simulink model "MainSim"  (R2024a)
settings: Solver=ode4  StartTime=0.0  StopTime=simtime  FixedStep=0.1  RelTol=1e-3
values from neighbouring files (symbols this model uses):
  C = [1 0 0 0 0 0 -1 0 0 0 0 0 ... (45 elements, 5x9)]    [C.mat]
undefined symbols (not defined in the file or in its folder): Ki, Kp, ssest, syys, utrim, xtrim
libraries: neural x680
(part 4 of 12)

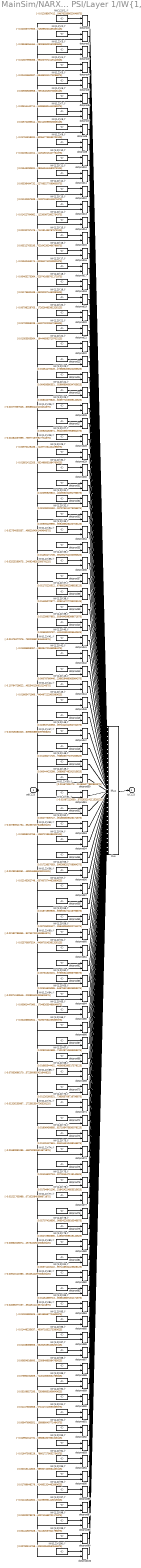
== system MainSim/NARX Controller NO PSI/Layer 1/IW{1,2} ==
  "pd{1,2}" : Inport  PortDimensions=5  SampleTime=0.1
      mask Display: e = 0.06;c1 = [120 230 180]/255;c2 = ([120 230 180]+0)/(256+128);c3 = ([120 230 180]+128)/(256+128);patch([0 1 1 0],[0 0 1 1],c1);patch([0 1 1 1-e 1-e 0+e],[0 0 1 1-e 0+e 0+e],c2);patch([0 0 1 1-e 0+e 0+e],[0 1 1 1-e 1-e 0+e],c3);plot([0 1 1 0 0],[0 0 1 1 0]);
  "IW{1,2}(1,:)'" : Constant  Value=[-0.012085674124014282593275737553994986228644847869873046875;-0.006873434973601206914028960426321646082215011119842529296875;-0.03332932307240245306534376368290395475924015045166015625;-0.03433322519643809689338098678490496240556240081787109375;0.030870812178684474413881133614268037490546703338623046875]
      mask Display: e = 0.06;c1 = [120 150 230]/255;c2 = ([120 150 230]+0)/383;c3 = ([120 150 230]+128)/383;patch([0 1 1 0],[0 0 1 1],c1);patch([0 1 1 1-e 1-e 0+e],[0 0 1 1-e 0+e 0+e],c2);patch([0 0 1 1-e 0+e 0+e],[0 1 1 1-e 1-e 0+e],c3);plot([0 1 1 0 0],[0 0 1 1 0]);disp('Weights');
  "IW{1,2}(10,:)'" : Constant  Value=[-0.022334120114864512707253396683881874196231365203857421875;0.03401133169790999943860043686072458513081073760986328125;-0.0140961839759349873146820897318320930935442447662353515625;-0.0105321300412540945490302846110353129915893077850341796875;0.0146962613745357205397024102921932353638112545013427734375]
      mask Display: e = 0.06;c1 = [120 150 230]/255;c2 = ([120 150 230]+0)/383;c3 = ([120 150 230]+128)/383;patch([0 1 1 0],[0 0 1 1],c1);patch([0 1 1 1-e 1-e 0+e],[0 0 1 1-e 0+e 0+e],c2);patch([0 0 1 1-e 0+e 0+e],[0 1 1 1-e 1-e 0+e],c3);plot([0 1 1 0 0],[0 0 1 1 0]);disp('Weights');
  "IW{1,2}(100,:)'" : Constant  Value=[0.007805117685184641100615277053975660237483680248260498046875;-0.016738192143750614537811571835845825262367725372314453125;0.0305525637743539746349341612585703842341899871826171875;0.02995618865728581770024874231239664368331432342529296875;-0.029207083950386396320464399423144641332328319549560546875]
      mask Display: e = 0.06;c1 = [120 150 230]/255;c2 = ([120 150 230]+0)/383;c3 = ([120 150 230]+128)/383;patch([0 1 1 0],[0 0 1 1],c1);patch([0 1 1 1-e 1-e 0+e],[0 0 1 1-e 0+e 0+e],c2);patch([0 0 1 1-e 0+e 0+e],[0 1 1 1-e 1-e 0+e],c3);plot([0 1 1 0 0],[0 0 1 1 0]);disp('Weights');
  "IW{1,2}(11,:)'" : Constant  Value=[0.0154329083187489911332956893375012441538274288177490234375;-0.022986085536823797070837827050127089023590087890625;0.024814779155320133841033936050735064782202243804931640625;0.0231971824718188550373820788763623568229377269744873046875;-0.0243675210208365751463066573023752425797283649444580078125]
      mask Display: e = 0.06;c1 = [120 150 230]/255;c2 = ([120 150 230]+0)/383;c3 = ([120 150 230]+128)/383;patch([0 1 1 0],[0 0 1 1],c1);patch([0 1 1 1-e 1-e 0+e],[0 0 1 1-e 0+e 0+e],c2);patch([0 0 1 1-e 0+e 0+e],[0 1 1 1-e 1-e 0+e],c3);plot([0 1 1 0 0],[0 0 1 1 0]);disp('Weights');
  "IW{1,2}(12,:)'" : Constant  Value=[0.005364947322163394170801975491258417605422437191009521484375;-0.0112431095377618119057760992518524290062487125396728515625;0.03357479632188732632247507581269019283354282379150390625;0.033744156754611308313140938253127387724816799163818359375;-0.031764486089429853910015566498259431682527065277099609375]
      mask Display: e = 0.06;c1 = [120 150 230]/255;c2 = ([120 150 230]+0)/383;c3 = ([120 150 230]+128)/383;patch([0 1 1 0],[0 0 1 1],c1);patch([0 1 1 1-e 1-e 0+e],[0 0 1 1-e 0+e 0+e],c2);patch([0 0 1 1-e 0+e 0+e],[0 1 1 1-e 1-e 0+e],c3);plot([0 1 1 0 0],[0 0 1 1 0]);disp('Weights');
  "IW{1,2}(13,:)'" : Constant  Value=[0.011323576395817040729507851892776670865714550018310546875;-0.0160785944939652557239551100565222441218793392181396484375;0.0287434696253211739713773198445778689347207546234130859375;0.0279514119935516079651360854541053413413465023040771484375;-0.0275897150154243812891774467743744025938212871551513671875]
      mask Display: e = 0.06;c1 = [120 150 230]/255;c2 = ([120 150 230]+0)/383;c3 = ([120 150 230]+128)/383;patch([0 1 1 0],[0 0 1 1],c1);patch([0 1 1 1-e 1-e 0+e],[0 0 1 1-e 0+e 0+e],c2);patch([0 0 1 1-e 0+e 0+e],[0 1 1 1-e 1-e 0+e],c3);plot([0 1 1 0 0],[0 0 1 1 0]);disp('Weights');
  "IW{1,2}(14,:)'" : Constant  Value=[-0.0142278498231365631288003470444891718216240406036376953125;-0.0098485858989617001968408516177078126929700374603271484375;-0.032202423742523557381733922966304817236959934234619140625;-0.03325848380519517977216281678920495323836803436279296875;0.029775514742350593644371059554032399319112300872802734375]
      mask Display: e = 0.06;c1 = [120 150 230]/255;c2 = ([120 150 230]+0)/383;c3 = ([120 150 230]+128)/383;patch([0 1 1 0],[0 0 1 1],c1);patch([0 1 1 1-e 1-e 0+e],[0 0 1 1-e 0+e 0+e],c2);patch([0 0 1 1-e 0+e 0+e],[0 1 1 1-e 1-e 0+e],c3);plot([0 1 1 0 0],[0 0 1 1 0]);disp('Weights');
  "IW{1,2}(15,:)'" : Constant  Value=[0.0223276747640495376590052956089493818581104278564453125;0.0284561503012705600823561979950682143680751323699951171875;0.02904798645340199436670758359468891285359859466552734375;0.0305503870117409294382415652080453583039343357086181640625;-0.0259989639895998880803063002531416714191436767578125]
      mask Display: e = 0.06;c1 = [120 150 230]/255;c2 = ([120 150 230]+0)/383;c3 = ([120 150 230]+128)/383;patch([0 1 1 0],[0 0 1 1],c1);patch([0 1 1 1-e 1-e 0+e],[0 0 1 1-e 0+e 0+e],c2);patch([0 0 1 1-e 0+e 0+e],[0 1 1 1-e 1-e 0+e],c3);plot([0 1 1 0 0],[0 0 1 1 0]);disp('Weights');
  "IW{1,2}(16,:)'" : Constant  Value=[0.005127631958366886399947048857939080335199832916259765625;0.00947650558097157778847385856124674319289624691009521484375;-0.0404557009729242522677594706692616455256938934326171875;-0.041547997688944203475980287976199178956449031829833984375;0.03786523265411989580542240219074301421642303466796875]
      mask Display: e = 0.06;c1 = [120 150 230]/255;c2 = ([120 150 230]+0)/383;c3 = ([120 150 230]+128)/383;patch([0 1 1 0],[0 0 1 1],c1);patch([0 1 1 1-e 1-e 0+e],[0 0 1 1-e 0+e 0+e],c2);patch([0 0 1 1-e 0+e 0+e],[0 1 1 1-e 1-e 0+e],c3);plot([0 1 1 0 0],[0 0 1 1 0]);disp('Weights');
  "IW{1,2}(17,:)'" : Constant  Value=[-0.0194245317476195757111501194458469399251043796539306640625;0.017930787047602224359987843627095571719110012054443359375;-0.01082284320194641484558228938794854911975562572479248046875;-0.009279432063260963092776734129074611701071262359619140625;0.01093748533229130064092782248508228803984820842742919921875]
      mask Display: e = 0.06;c1 = [120 150 230]/255;c2 = ([120 150 230]+0)/383;c3 = ([120 150 230]+128)/383;patch([0 1 1 0],[0 0 1 1],c1);patch([0 1 1 1-e 1-e 0+e],[0 0 1 1-e 0+e 0+e],c2);patch([0 0 1 1-e 0+e 0+e],[0 1 1 1-e 1-e 0+e],c3);plot([0 1 1 0 0],[0 0 1 1 0]);disp('Weights');
  "IW{1,2}(18,:)'" : Constant  Value=[-0.004632733645585514724307696354799190885387361049652099609375;0.038132997508550599274901315993702155537903308868408203125;-0.027774570134460885295624166246852837502956390380859375;-0.0258087635385522186359796847909819916822016239166259765625;0.0275425986452899444756337032913506845943629741668701171875]
      mask Display: e = 0.06;c1 = [120 150 230]/255;c2 = ([120 150 230]+0)/383;c3 = ([120 150 230]+128)/383;patch([0 1 1 0],[0 0 1 1],c1);patch([0 1 1 1-e 1-e 0+e],[0 0 1 1-e 0+e 0+e],c2);patch([0 0 1 1-e 0+e 0+e],[0 1 1 1-e 1-e 0+e],c3);plot([0 1 1 0 0],[0 0 1 1 0]);disp('Weights');
  "IW{1,2}(19,:)'" : Constant  Value=[0.0117563243958725520410535381188310566358268260955810546875;0.0199784928711961538849717356924884370528161525726318359375;0.035521756938338443221336859778602956794202327728271484375;0.037526953635152134058916573167152819223701953887939453125;-0.032272748785357442680155060088509344495832920074462890625]
      mask Display: e = 0.06;c1 = [120 150 230]/255;c2 = ([120 150 230]+0)/383;c3 = ([120 150 230]+128)/383;patch([0 1 1 0],[0 0 1 1],c1);patch([0 1 1 1-e 1-e 0+e],[0 0 1 1-e 0+e 0+e],c2);patch([0 0 1 1-e 0+e 0+e],[0 1 1 1-e 1-e 0+e],c3);plot([0 1 1 0 0],[0 0 1 1 0]);disp('Weights');
  "IW{1,2}(2,:)'" : Constant  Value=[-0.020337079051551763819727369764223112724721431732177734375;0.0017909882428626361199064387363932837615720927715301513671875;-0.0259369100125725615679783686573500744998455047607421875;-0.02554043369616378067465944923242204822599887847900390625;0.024521120571637362861583397943832096643745899200439453125]
      mask Display: e = 0.06;c1 = [120 150 230]/255;c2 = ([120 150 230]+0)/383;c3 = ([120 150 230]+128)/383;patch([0 1 1 0],[0 0 1 1],c1);patch([0 1 1 1-e 1-e 0+e],[0 0 1 1-e 0+e 0+e],c2);patch([0 0 1 1-e 0+e 0+e],[0 1 1 1-e 1-e 0+e],c3);plot([0 1 1 0 0],[0 0 1 1 0]);disp('Weights');
  "IW{1,2}(20,:)'" : Constant  Value=[-0.00798228763147881305306530208554249838925898075103759765625;0.0261395622475988458066620268027691054157912731170654296875;-0.0273294398816671772756148328653580392710864543914794921875;-0.0260723881186434407186691686320045846514403820037841796875;0.0266414429954283833723582830543819000013172626495361328125]
      mask Display: e = 0.06;c1 = [120 150 230]/255;c2 = ([120 150 230]+0)/383;c3 = ([120 150 230]+128)/383;patch([0 1 1 0],[0 0 1 1],c1);patch([0 1 1 1-e 1-e 0+e],[0 0 1 1-e 0+e 0+e],c2);patch([0 0 1 1-e 0+e 0+e],[0 1 1 1-e 1-e 0+e],c3);plot([0 1 1 0 0],[0 0 1 1 0]);disp('Weights');
  "IW{1,2}(21,:)'" : Constant  Value=[0.0170095923909163726506221792078576982021331787109375;0.0187237871314250119147981621381404693238437175750732421875;0.03149959520865823481283740647995728068053722381591796875;0.032961086247749522837313662648739409632980823516845703125;-0.0287231551207946245174440491609857417643070220947265625]
      mask Display: e = 0.06;c1 = [120 150 230]/255;c2 = ([120 150 230]+0)/383;c3 = ([120 150 230]+128)/383;patch([0 1 1 0],[0 0 1 1],c1);patch([0 1 1 1-e 1-e 0+e],[0 0 1 1-e 0+e 0+e],c2);patch([0 0 1 1-e 0+e 0+e],[0 1 1 1-e 1-e 0+e],c3);plot([0 1 1 0 0],[0 0 1 1 0]);disp('Weights');
  "IW{1,2}(22,:)'" : Constant  Value=[0.010535055642576562906498338634264655411243438720703125;0.01042574641511804893478920774896323564462363719940185546875;0.034974439983853473912223108754915301688015460968017578125;0.036382770125930108395806428234209306538105010986328125;-0.032197350517627738863968289706463110633194446563720703125]
      mask Display: e = 0.06;c1 = [120 150 230]/255;c2 = ([120 150 230]+0)/383;c3 = ([120 150 230]+128)/383;patch([0 1 1 0],[0 0 1 1],c1);patch([0 1 1 1-e 1-e 0+e],[0 0 1 1-e 0+e 0+e],c2);patch([0 0 1 1-e 0+e 0+e],[0 1 1 1-e 1-e 0+e],c3);plot([0 1 1 0 0],[0 0 1 1 0]);disp('Weights');
  "IW{1,2}(23,:)'" : Constant  Value=[0.01054470049731781773616479114252797444351017475128173828125;-0.003714267250142730576734084735335272853262722492218017578125;0.031988890860725600895353437636003945954144001007080078125;0.032309519654246325603974554496744531206786632537841796875;-0.030067687396656585241405679198578582145273685455322265625]
      mask Display: e = 0.06;c1 = [120 150 230]/255;c2 = ([120 150 230]+0)/383;c3 = ([120 150 230]+128)/383;patch([0 1 1 0],[0 0 1 1],c1);patch([0 1 1 1-e 1-e 0+e],[0 0 1 1-e 0+e 0+e],c2);patch([0 0 1 1-e 0+e 0+e],[0 1 1 1-e 1-e 0+e],c3);plot([0 1 1 0 0],[0 0 1 1 0]);disp('Weights');
  "IW{1,2}(24,:)'" : Constant  Value=[0.004595803517489915369920172594220275641418993473052978515625;-0.003429596191471447237664182949856694904156029224395751953125;0.03579031809052179990970898870727978646755218505859375;0.036524311932395726876254826720469282008707523345947265625;-0.0334344069763509443848903401885763742029666900634765625]
      mask Display: e = 0.06;c1 = [120 150 230]/255;c2 = ([120 150 230]+0)/383;c3 = ([120 150 230]+128)/383;patch([0 1 1 0],[0 0 1 1],c1);patch([0 1 1 1-e 1-e 0+e],[0 0 1 1-e 0+e 0+e],c2);patch([0 0 1 1-e 0+e 0+e],[0 1 1 1-e 1-e 0+e],c3);plot([0 1 1 0 0],[0 0 1 1 0]);disp('Weights');
  "IW{1,2}(25,:)'" : Constant  Value=[0.00804079845644819525551927341666669235564768314361572265625;0.027652292619962597075566890225672977976500988006591796875;0.0393458565658561243427726594745763577520847320556640625;0.0420552906947410376492513250923366285860538482666015625;-0.035294613228765016332832971102106967009603977203369140625]
      mask Display: e = 0.06;c1 = [120 150 230]/255;c2 = ([120 150 230]+0)/383;c3 = ([120 150 230]+128)/383;patch([0 1 1 0],[0 0 1 1],c1);patch([0 1 1 1-e 1-e 0+e],[0 0 1 1-e 0+e 0+e],c2);patch([0 0 1 1-e 0+e 0+e],[0 1 1 1-e 1-e 0+e],c3);plot([0 1 1 0 0],[0 0 1 1 0]);disp('Weights');
  "IW{1,2}(26,:)'" : Constant  Value=[-0.015778575262286022307112176576993078924715518951416015625;-0.016297336723622379839326868022908456623554229736328125;-0.03222094803741291924037426497307023964822292327880859375;-0.033707220692914575954635125754066393710672855377197265625;0.0293691191872800204387683464801739319227635860443115234375]
      mask Display: e = 0.06;c1 = [120 150 230]/255;c2 = ([120 150 230]+0)/383;c3 = ([120 150 230]+128)/383;patch([0 1 1 0],[0 0 1 1],c1);patch([0 1 1 1-e 1-e 0+e],[0 0 1 1-e 0+e 0+e],c2);patch([0 0 1 1-e 0+e 0+e],[0 1 1 1-e 1-e 0+e],c3);plot([0 1 1 0 0],[0 0 1 1 0]);disp('Weights');
  "IW{1,2}(27,:)'" : Constant  Value=[0.0092646367179257359258937043477999395690858364105224609375;-0.002664960154736236049022313210343781975097954273223876953125;0.033000129533506929180308731019977130927145481109619140625;0.033420340489081011570160484325242578051984310150146484375;-0.03090370828399358060778467915952205657958984375]
      mask Display: e = 0.06;c1 = [120 150 230]/255;c2 = ([120 150 230]+0)/383;c3 = ([120 150 230]+128)/383;patch([0 1 1 0],[0 0 1 1],c1);patch([0 1 1 1-e 1-e 0+e],[0 0 1 1-e 0+e 0+e],c2);patch([0 0 1 1-e 0+e 0+e],[0 1 1 1-e 1-e 0+e],c3);plot([0 1 1 0 0],[0 0 1 1 0]);disp('Weights');
  "IW{1,2}(28,:)'" : Constant  Value=[-0.0108403789940856552787007416327469400130212306976318359375;-0.017317287252119110962933490327486651949584484100341796875;-0.03607743082670518408594517723031458444893360137939453125;-0.0379691018103407440520413729245774447917938232421875;0.03292014375354500310688621311783208511769771575927734375]
      mask Display: e = 0.06;c1 = [120 150 230]/255;c2 = ([120 150 230]+0)/383;c3 = ([120 150 230]+128)/383;patch([0 1 1 0],[0 0 1 1],c1);patch([0 1 1 1-e 1-e 0+e],[0 0 1 1-e 0+e 0+e],c2);patch([0 0 1 1-e 0+e 0+e],[0 1 1 1-e 1-e 0+e],c3);plot([0 1 1 0 0],[0 0 1 1 0]);disp('Weights');
  "IW{1,2}(29,:)'" : Constant  Value=[-0.00970129436445513367026638462675691698677837848663330078125;-0.007632062964286630800392341456017675227485597133636474609375;-0.034895110867124011500006730557288392446935176849365234375;-0.036176316847200296056286106249899603426456451416015625;0.032250133329590473241221815214885282330214977264404296875]
      mask Display: e = 0.06;c1 = [120 150 230]/255;c2 = ([120 150 230]+0)/383;c3 = ([120 150 230]+128)/383;patch([0 1 1 0],[0 0 1 1],c1);patch([0 1 1 1-e 1-e 0+e],[0 0 1 1-e 0+e 0+e],c2);patch([0 0 1 1-e 0+e 0+e],[0 1 1 1-e 1-e 0+e],c3);plot([0 1 1 0 0],[0 0 1 1 0]);disp('Weights');
  "IW{1,2}(3,:)'" : Constant  Value=[-0.035362644649990004896977779935696162283420562744140625;0.0034190428224744641438892500673318863846361637115478515625;-0.0164693714271560709416775125646381638944149017333984375;-0.01521402214412888830030734510501133627258241176605224609375;0.0163416210479518132780984984719907515682280063629150390625]
      mask Display: e = 0.06;c1 = [120 150 230]/255;c2 = ([120 150 230]+0)/383;c3 = ([120 150 230]+128)/383;patch([0 1 1 0],[0 0 1 1],c1);patch([0 1 1 1-e 1-e 0+e],[0 0 1 1-e 0+e 0+e],c2);patch([0 0 1 1-e 0+e 0+e],[0 1 1 1-e 1-e 0+e],c3);plot([0 1 1 0 0],[0 0 1 1 0]);disp('Weights');
  "IW{1,2}(30,:)'" : Constant  Value=[-0.0185141220369085569841249849787345738150179386138916015625;-0.019445746310621014885100521496497094631195068359375;-0.03028812136673748878212819590771687217056751251220703125;-0.031649523029389219075380168533229152671992778778076171875;0.027495729389122515462506868288983241654932498931884765625]
      mask Display: e = 0.06;c1 = [120 150 230]/255;c2 = ([120 150 230]+0)/383;c3 = ([120 150 230]+128)/383;patch([0 1 1 0],[0 0 1 1],c1);patch([0 1 1 1-e 1-e 0+e],[0 0 1 1-e 0+e 0+e],c2);patch([0 0 1 1-e 0+e 0+e],[0 1 1 1-e 1-e 0+e],c3);plot([0 1 1 0 0],[0 0 1 1 0]);disp('Weights');
  "IW{1,2}(31,:)'" : Constant  Value=[0.0209592981063579930633977710385806858539581298828125;0.01083804268023169474488565100500636617653071880340576171875;0.02844881735902089758827315790767897851765155792236328125;0.0289792660465030722793944306658886489458382129669189453125;-0.0263099639549649981506984630641454714350402355194091796875]
      mask Display: e = 0.06;c1 = [120 150 230]/255;c2 = ([120 150 230]+0)/383;c3 = ([120 150 230]+128)/383;patch([0 1 1 0],[0 0 1 1],c1);patch([0 1 1 1-e 1-e 0+e],[0 0 1 1-e 0+e 0+e],c2);patch([0 0 1 1-e 0+e 0+e],[0 1 1 1-e 1-e 0+e],c3);plot([0 1 1 0 0],[0 0 1 1 0]);disp('Weights');
  "IW{1,2}(32,:)'" : Constant  Value=[0.00109203150034972739680638742498786086798645555973052978515625;-0.03211495284359179580579990442856797017157077789306640625;0.02263060499647796819377987276311614550650119781494140625;0.0217302598444287509149575043920776806771755218505859375;-0.022336808035550263784596580762809026055037975311279296875]
      mask Display: e = 0.06;c1 = [120 150 230]/255;c2 = ([120 150 230]+0)/383;c3 = ([120 150 230]+128)/383;patch([0 1 1 0],[0 0 1 1],c1);patch([0 1 1 1-e 1-e 0+e],[0 0 1 1-e 0+e 0+e],c2);patch([0 0 1 1-e 0+e 0+e],[0 1 1 1-e 1-e 0+e],c3);plot([0 1 1 0 0],[0 0 1 1 0]);disp('Weights');
  "IW{1,2}(33,:)'" : Constant  Value=[0.009394299901924745010983741622112574987113475799560546875;0.01240127959912632783778807521457565599121153354644775390625;0.035979459082758201426965882774311467073857784271240234375;0.037457031953582069216945882317304494790732860565185546875;-0.032943621454636924650305473960543167777359485626220703125]
      mask Display: e = 0.06;c1 = [120 150 230]/255;c2 = ([120 150 230]+0)/383;c3 = ([120 150 230]+128)/383;patch([0 1 1 0],[0 0 1 1],c1);patch([0 1 1 1-e 1-e 0+e],[0 0 1 1-e 0+e 0+e],c2);patch([0 0 1 1-e 0+e 0+e],[0 1 1 1-e 1-e 0+e],c3);plot([0 1 1 0 0],[0 0 1 1 0]);disp('Weights');
  "IW{1,2}(34,:)'" : Constant  Value=[-0.0275405033706076669830498104829530348069965839385986328125;0.0703696860545029168054753654359956271946430206298828125;0.005069886952264021119651804525574334547854959964752197265625;0.01091440888194798730648216178451548330485820770263671875;-0.000748953531080119561634533820182468843995593488216400146484375]
      mask Display: e = 0.06;c1 = [120 150 230]/255;c2 = ([120 150 230]+0)/383;c3 = ([120 150 230]+128)/383;patch([0 1 1 0],[0 0 1 1],c1);patch([0 1 1 1-e 1-e 0+e],[0 0 1 1-e 0+e 0+e],c2);patch([0 0 1 1-e 0+e 0+e],[0 1 1 1-e 1-e 0+e],c3);plot([0 1 1 0 0],[0 0 1 1 0]);disp('Weights');
  "IW{1,2}(35,:)'" : Constant  Value=[0.01450471706758239311130243009984042146243155002593994140625;0.0097224222835883729321171387027789023704826831817626953125;0.0318943988301988168299061499055824242532253265380859375;0.032828070117499698332697022351567284204065799713134765625;-0.0294356770008160940899077928634142153896391391754150390625]
      mask Display: e = 0.06;c1 = [120 150 230]/255;c2 = ([120 150 230]+0)/383;c3 = ([120 150 230]+128)/383;patch([0 1 1 0],[0 0 1 1],c1);patch([0 1 1 1-e 1-e 0+e],[0 0 1 1-e 0+e 0+e],c2);patch([0 0 1 1-e 0+e 0+e],[0 1 1 1-e 1-e 0+e],c3);plot([0 1 1 0 0],[0 0 1 1 0]);disp('Weights');
  "IW{1,2}(36,:)'" : Constant  Value=[-0.0252526907569290415267460048198699951171875;0.006006617520969024549837289583820165717042982578277587890625;-0.0222568762548918976096334887415650882758200168609619140625;-0.021182460559284639611821177140882355161011219024658203125;0.0214335734412836771689558901243799482472240924835205078125]
      mask Display: e = 0.06;c1 = [120 150 230]/255;c2 = ([120 150 230]+0)/383;c3 = ([120 150 230]+128)/383;patch([0 1 1 0],[0 0 1 1],c1);patch([0 1 1 1-e 1-e 0+e],[0 0 1 1-e 0+e 0+e],c2);patch([0 0 1 1-e 0+e 0+e],[0 1 1 1-e 1-e 0+e],c3);plot([0 1 1 0 0],[0 0 1 1 0]);disp('Weights');
  "IW{1,2}(37,:)'" : Constant  Value=[0.02175220512435248332305803842245950363576412200927734375;-0.00682407870694965064395365317295727436430752277374267578125;0.0233296889759175181400241427809305605478584766387939453125;0.022841356027361113534279724035513936541974544525146484375;-0.022426131421705526591825474724828382022678852081298828125]
      mask Display: e = 0.06;c1 = [120 150 230]/255;c2 = ([120 150 230]+0)/383;c3 = ([120 150 230]+128)/383;patch([0 1 1 0],[0 0 1 1],c1);patch([0 1 1 1-e 1-e 0+e],[0 0 1 1-e 0+e 0+e],c2);patch([0 0 1 1-e 0+e 0+e],[0 1 1 1-e 1-e 0+e],c3);plot([0 1 1 0 0],[0 0 1 1 0]);disp('Weights');
  "IW{1,2}(38,:)'" : Constant  Value=[0.0143507097716770760931215278333183960057795047760009765625;0.0269671999261726913488246282213367521762847900390625;0.0353867336342915950186949203271069563925266265869140625;0.0373802734921193924311211276290123350918292999267578125;-0.0316924028888075082210917798875016160309314727783203125]
      mask Display: e = 0.06;c1 = [120 150 230]/255;c2 = ([120 150 230]+0)/383;c3 = ([120 150 230]+128)/383;patch([0 1 1 0],[0 0 1 1],c1);patch([0 1 1 1-e 1-e 0+e],[0 0 1 1-e 0+e 0+e],c2);patch([0 0 1 1-e 0+e 0+e],[0 1 1 1-e 1-e 0+e],c3);plot([0 1 1 0 0],[0 0 1 1 0]);disp('Weights');
  "IW{1,2}(39,:)'" : Constant  Value=[0.0123990788148799040147007843870596843771636486053466796875;0.01315418727855812049132300245446458575315773487091064453125;0.034021033735004597986506524875949253328144550323486328125;0.035401007196237004037708828718677978031337261199951171875;-0.03119892993377297585322338591140578500926494598388671875]
      mask Display: e = 0.06;c1 = [120 150 230]/255;c2 = ([120 150 230]+0)/383;c3 = ([120 150 230]+128)/383;patch([0 1 1 0],[0 0 1 1],c1);patch([0 1 1 1-e 1-e 0+e],[0 0 1 1-e 0+e 0+e],c2);patch([0 0 1 1-e 0+e 0+e],[0 1 1 1-e 1-e 0+e],c3);plot([0 1 1 0 0],[0 0 1 1 0]);disp('Weights');
  "IW{1,2}(4,:)'" : Constant  Value=[-0.01307995066120812809040696578222195967100560665130615234375;-0.005244252812554919644660866850927050109021365642547607421875;-0.0322158939167921654078696747092180885374546051025390625;-0.0329942700597006532969857062198570929467678070068359375;0.0299180848159462421664844811175498762167990207672119140625]
      mask Display: e = 0.06;c1 = [120 150 230]/255;c2 = ([120 150 230]+0)/383;c3 = ([120 150 230]+128)/383;patch([0 1 1 0],[0 0 1 1],c1);patch([0 1 1 1-e 1-e 0+e],[0 0 1 1-e 0+e 0+e],c2);patch([0 0 1 1-e 0+e 0+e],[0 1 1 1-e 1-e 0+e],c3);plot([0 1 1 0 0],[0 0 1 1 0]);disp('Weights');
  "IW{1,2}(40,:)'" : Constant  Value=[0.005830297976655092646869338324222553637810051441192626953125;-0.032969565421287476414402561886163312010467052459716796875;0.02701713372407664459640130871775909326970577239990234375;0.0253605387684672257953000240604524151422083377838134765625;-0.026580191374984997454422597229495295323431491851806640625]
      mask Display: e = 0.06;c1 = [120 150 230]/255;c2 = ([120 150 230]+0)/383;c3 = ([120 150 230]+128)/383;patch([0 1 1 0],[0 0 1 1],c1);patch([0 1 1 1-e 1-e 0+e],[0 0 1 1-e 0+e 0+e],c2);patch([0 0 1 1-e 0+e 0+e],[0 1 1 1-e 1-e 0+e],c3);plot([0 1 1 0 0],[0 0 1 1 0]);disp('Weights');
  "IW{1,2}(41,:)'" : Constant  Value=[-0.024753779764514420580479026057219016365706920623779296875;0.035539965068515776136504058513310155831277370452880859375;-0.015747777853394047398172261864601750858128070831298828125;-0.01329751468211923075279923267544290865771472454071044921875;0.0170777252142555978353666290558976470492780208587646484375]
      mask Display: e = 0.06;c1 = [120 150 230]/255;c2 = ([120 150 230]+0)/383;c3 = ([120 150 230]+128)/383;patch([0 1 1 0],[0 0 1 1],c1);patch([0 1 1 1-e 1-e 0+e],[0 0 1 1-e 0+e 0+e],c2);patch([0 0 1 1-e 0+e 0+e],[0 1 1 1-e 1-e 0+e],c3);plot([0 1 1 0 0],[0 0 1 1 0]);disp('Weights');
  "IW{1,2}(42,:)'" : Constant  Value=[-0.0138585905799956284056850819297324051149189472198486328125;0.0222236545812980988701124118733787327073514461517333984375;-0.025691349558800681551762323806542553938925266265869140625;-0.0242299867515220757052674116494017653167247772216796875;0.02508107576127059645809680432648747228085994720458984375]
      mask Display: e = 0.06;c1 = [120 150 230]/255;c2 = ([120 150 230]+0)/383;c3 = ([120 150 230]+128)/383;patch([0 1 1 0],[0 0 1 1],c1);patch([0 1 1 1-e 1-e 0+e],[0 0 1 1-e 0+e 0+e],c2);patch([0 0 1 1-e 0+e 0+e],[0 1 1 1-e 1-e 0+e],c3);plot([0 1 1 0 0],[0 0 1 1 0]);disp('Weights');
  "IW{1,2}(43,:)'" : Constant  Value=[0.00078766446852296888823941056756439138553105294704437255859375;-0.01318593236706018523296535249755834229290485382080078125;0.035554632787187519238347732652982813306152820587158203125;0.035671472005832323415308593439476680941879749298095703125;-0.03350454338703233447827045665690093301236629486083984375]
      mask Display: e = 0.06;c1 = [120 150 230]/255;c2 = ([120 150 230]+0)/383;c3 = ([120 150 230]+128)/383;patch([0 1 1 0],[0 0 1 1],c1);patch([0 1 1 1-e 1-e 0+e],[0 0 1 1-e 0+e 0+e],c2);patch([0 0 1 1-e 0+e 0+e],[0 1 1 1-e 1-e 0+e],c3);plot([0 1 1 0 0],[0 0 1 1 0]);disp('Weights');
  "IW{1,2}(44,:)'" : Constant  Value=[-0.10794728622973730203238318381409044377505779266357421875;0.080654689400765422480077404543408192694187164306640625;-0.006712287955641473881363001652289312914945185184478759765625;-0.00470443324641543932085330226300357026048004627227783203125;0.016195459593009574328359434502999647520482540130615234375]
      mask Display: e = 0.06;c1 = [120 150 230]/255;c2 = ([120 150 230]+0)/383;c3 = ([120 150 230]+128)/383;patch([0 1 1 0],[0 0 1 1],c1);patch([0 1 1 1-e 1-e 0+e],[0 0 1 1-e 0+e 0+e],c2);patch([0 0 1 1-e 0+e 0+e],[0 1 1 1-e 1-e 0+e],c3);plot([0 1 1 0 0],[0 0 1 1 0]);disp('Weights');
  "IW{1,2}(45,:)'" : Constant  Value=[-0.0166547196653716624015206804187982925213873386383056640625;-0.021930555020089163853480584975841338746249675750732421875;-0.03235377835425763681787003633871790952980518341064453125;-0.033854060228525099940366516193535062484443187713623046875;0.029165569951700033579644610881587141193449497222900390625]
      mask Display: e = 0.06;c1 = [120 150 230]/255;c2 = ([120 150 230]+0)/383;c3 = ([120 150 230]+128)/383;patch([0 1 1 0],[0 0 1 1],c1);patch([0 1 1 1-e 1-e 0+e],[0 0 1 1-e 0+e 0+e],c2);patch([0 0 1 1-e 0+e 0+e],[0 1 1 1-e 1-e 0+e],c3);plot([0 1 1 0 0],[0 0 1 1 0]);disp('Weights');
  "IW{1,2}(46,:)'" : Constant  Value=[0.0235374635883499293276255315277012414298951625823974609375;-0.0253972895783901343735866618089858093298971652984619140625;0.01196160632864553576004684742883910075761377811431884765625;0.0089294032274018948769356285311005194671452045440673828125;-0.0122044634295307395654983650956637575291097164154052734375]
      mask Display: e = 0.06;c1 = [120 150 230]/255;c2 = ([120 150 230]+0)/383;c3 = ([120 150 230]+128)/383;patch([0 1 1 0],[0 0 1 1],c1);patch([0 1 1 1-e 1-e 0+e],[0 0 1 1-e 0+e 0+e],c2);patch([0 0 1 1-e 0+e 0+e],[0 1 1 1-e 1-e 0+e],c3);plot([0 1 1 0 0],[0 0 1 1 0]);disp('Weights');
  "IW{1,2}(47,:)'" : Constant  Value=[-0.0191508162319503905113293740214430727064609527587890625;0.018575161632503965625229369607041007839143276214599609375;-0.02135301021187473169415937945814221166074275970458984375;-0.020013423739152387537121313698662561364471912384033203125;0.021090343821238678734264482272919849492609500885009765625]
      mask Display: e = 0.06;c1 = [120 150 230]/255;c2 = ([120 150 230]+0)/383;c3 = ([120 150 230]+128)/383;patch([0 1 1 0],[0 0 1 1],c1);patch([0 1 1 1-e 1-e 0+e],[0 0 1 1-e 0+e 0+e],c2);patch([0 0 1 1-e 0+e 0+e],[0 1 1 1-e 1-e 0+e],c3);plot([0 1 1 0 0],[0 0 1 1 0]);disp('Weights');
  "IW{1,2}(48,:)'" : Constant  Value=[0.01108471725165885955755040725989601924084126949310302734375;0.00499202294705096243088160434808742138557136058807373046875;0.03323706194139654235275571636520908214151859283447265625;0.034128203303954225689142987221202929504215717315673828125;-0.0307945443921934271236384716985412524081766605377197265625]
      mask Display: e = 0.06;c1 = [120 150 230]/255;c2 = ([120 150 230]+0)/383;c3 = ([120 150 230]+128)/383;patch([0 1 1 0],[0 0 1 1],c1);patch([0 1 1 1-e 1-e 0+e],[0 0 1 1-e 0+e 0+e],c2);patch([0 0 1 1-e 0+e 0+e],[0 1 1 1-e 1-e 0+e],c3);plot([0 1 1 0 0],[0 0 1 1 0]);disp('Weights');
  "IW{1,2}(49,:)'" : Constant  Value=[0.000444232882168411695976428799070845343521796166896820068359375;0.007147187728769891813807024760762942605651915073394775390625;0.04011494478521133999482373155842651613056659698486328125;0.042136968623270994183105386809984338469803333282470703125;-0.036877481948935177114012873289539129473268985748291015625]
      mask Display: e = 0.06;c1 = [120 150 230]/255;c2 = ([120 150 230]+0)/383;c3 = ([120 150 230]+128)/383;patch([0 1 1 0],[0 0 1 1],c1);patch([0 1 1 1-e 1-e 0+e],[0 0 1 1-e 0+e 0+e],c2);patch([0 0 1 1-e 0+e 0+e],[0 1 1 1-e 1-e 0+e],c3);plot([0 1 1 0 0],[0 0 1 1 0]);disp('Weights');
  "IW{1,2}(5,:)'" : Constant  Value=[-0.0243166293786484070948983315929581294767558574676513671875;-0.042345698652544568052480400410786387510597705841064453125;-0.031002494159611586332925270426130737178027629852294921875;-0.032776692733758792941411996935130446217954158782958984375;0.026827756970903837707709271853673271834850311279296875]
      mask Display: e = 0.06;c1 = [120 150 230]/255;c2 = ([120 150 230]+0)/383;c3 = ([120 150 230]+128)/383;patch([0 1 1 0],[0 0 1 1],c1);patch([0 1 1 1-e 1-e 0+e],[0 0 1 1-e 0+e 0+e],c2);patch([0 0 1 1-e 0+e 0+e],[0 1 1 1-e 1-e 0+e],c3);plot([0 1 1 0 0],[0 0 1 1 0]);disp('Weights');
  "IW{1,2}(50,:)'" : Constant  Value=[0.015679052731908484086265076484778546728193759918212890625;0.019820006965748794558468404147788533009588718414306640625;0.032860845027851061372903274104828597046434879302978515625;0.03431681907809210063664551171314087696373462677001953125;-0.0297726735613363067967096498023238382302224636077880859375]
      mask Display: e = 0.06;c1 = [120 150 230]/255;c2 = ([120 150 230]+0)/383;c3 = ([120 150 230]+128)/383;patch([0 1 1 0],[0 0 1 1],c1);patch([0 1 1 1-e 1-e 0+e],[0 0 1 1-e 0+e 0+e],c2);patch([0 0 1 1-e 0+e 0+e],[0 1 1 1-e 1-e 0+e],c3);plot([0 1 1 0 0],[0 0 1 1 0]);disp('Weights');
  "IW{1,2}(51,:)'" : Constant  Value=[-0.0108721265074406929496131368750866386108100414276123046875;-0.01997518134507371423413957245429628528654575347900390625;-0.03596314530959342226079655802095658145844936370849609375;-0.03788649806996369218126119449152611196041107177734375;0.032598422850122432681274631249834783375263214111328125]
      mask Display: e = 0.06;c1 = [120 150 230]/255;c2 = ([120 150 230]+0)/383;c3 = ([120 150 230]+128)/383;patch([0 1 1 0],[0 0 1 1],c1);patch([0 1 1 1-e 1-e 0+e],[0 0 1 1-e 0+e 0+e],c2);patch([0 0 1 1-e 0+e 0+e],[0 1 1 1-e 1-e 0+e],c3);plot([0 1 1 0 0],[0 0 1 1 0]);disp('Weights');
  "IW{1,2}(52,:)'" : Constant  Value=[0.0027730574770842321419284104422331438399851322174072265625;-0.0162628923088370160032756217560745426453649997711181640625;0.033927117272200220388089775269691017456352710723876953125;0.03376892068720492579014802458914346061646938323974609375;-0.032196559291150887716081996359207550995051860809326171875]
      mask Display: e = 0.06;c1 = [120 150 230]/255;c2 = ([120 150 230]+0)/383;c3 = ([120 150 230]+128)/383;patch([0 1 1 0],[0 0 1 1],c1);patch([0 1 1 1-e 1-e 0+e],[0 0 1 1-e 0+e 0+e],c2);patch([0 0 1 1-e 0+e 0+e],[0 1 1 1-e 1-e 0+e],c3);plot([0 1 1 0 0],[0 0 1 1 0]);disp('Weights');
  "IW{1,2}(53,:)'" : Constant  Value=[-0.0078391175469601261094343414015384041704237461090087890625;0.034706112228070483405328872095196857117116451263427734375;-0.024505097646106692443890295862729544751346111297607421875;-0.022330097231736574514560089710357715375721454620361328125;0.02425963908850647943182821109076030552387237548828125]
      mask Display: e = 0.06;c1 = [120 150 230]/255;c2 = ([120 150 230]+0)/383;c3 = ([120 150 230]+128)/383;patch([0 1 1 0],[0 0 1 1],c1);patch([0 1 1 1-e 1-e 0+e],[0 0 1 1-e 0+e 0+e],c2);patch([0 0 1 1-e 0+e 0+e],[0 1 1 1-e 1-e 0+e],c3);plot([0 1 1 0 0],[0 0 1 1 0]);disp('Weights');
  "IW{1,2}(54,:)'" : Constant  Value=[-0.0185931276607731628403019641382343252189457416534423828125;0.04198174271007330815574931648370693437755107879638671875;-0.060929311059334252675956378197952290065586566925048828125;-0.0640894246806532896787444997244165278971195220947265625;0.057302211087786721066539286084662307985126972198486328125]
      mask Display: e = 0.06;c1 = [120 150 230]/255;c2 = ([120 150 230]+0)/383;c3 = ([120 150 230]+128)/383;patch([0 1 1 0],[0 0 1 1],c1);patch([0 1 1 1-e 1-e 0+e],[0 0 1 1-e 0+e 0+e],c2);patch([0 0 1 1-e 0+e 0+e],[0 1 1 1-e 1-e 0+e],c3);plot([0 1 1 0 0],[0 0 1 1 0]);disp('Weights');
  "IW{1,2}(55,:)'" : Constant  Value=[0.0172365708330581395013592072018582257442176342010498046875;-0.042219484639421711591467101243324577808380126953125;0.0200781206626008401627814237144775688648223876953125;0.0165276686536828358586870280078073847107589244842529296875;-0.021198751002557379707891271891639917157590389251708984375]
      mask Display: e = 0.06;c1 = [120 150 230]/255;c2 = ([120 150 230]+0)/383;c3 = ([120 150 230]+128)/383;patch([0 1 1 0],[0 0 1 1],c1);patch([0 1 1 1-e 1-e 0+e],[0 0 1 1-e 0+e 0+e],c2);patch([0 0 1 1-e 0+e 0+e],[0 1 1 1-e 1-e 0+e],c3);plot([0 1 1 0 0],[0 0 1 1 0]);disp('Weights');
  "IW{1,2}(56,:)'" : Constant  Value=[-0.01299183061693336312114599451206231606192886829376220703125;-0.0095734824668631361699322468439277145080268383026123046875;-0.0325962528791546024553582583394018001854419708251953125;-0.033530968212940270856137203736579976975917816162109375;0.0299594111131194947017508667386209708638489246368408203125]
      mask Display: e = 0.06;c1 = [120 150 230]/255;c2 = ([120 150 230]+0)/383;c3 = ([120 150 230]+128)/383;patch([0 1 1 0],[0 0 1 1],c1);patch([0 1 1 1-e 1-e 0+e],[0 0 1 1-e 0+e 0+e],c2);patch([0 0 1 1-e 0+e 0+e],[0 1 1 1-e 1-e 0+e],c3);plot([0 1 1 0 0],[0 0 1 1 0]);disp('Weights');
  "IW{1,2}(57,:)'" : Constant  Value=[-0.0214530274965023248778805964320781640708446502685546875;-0.058368613447681995387572584377267048694193363189697265625;-0.03772837533167784640486530634007067419588565826416015625;-0.042649015920922461742037512522074393928050994873046875;0.03275698016424179181971254593008779920637607574462890625]
      mask Display: e = 0.06;c1 = [120 150 230]/255;c2 = ([120 150 230]+0)/383;c3 = ([120 150 230]+128)/383;patch([0 1 1 0],[0 0 1 1],c1);patch([0 1 1 1-e 1-e 0+e],[0 0 1 1-e 0+e 0+e],c2);patch([0 0 1 1-e 0+e 0+e],[0 1 1 1-e 1-e 0+e],c3);plot([0 1 1 0 0],[0 0 1 1 0]);disp('Weights');
  "IW{1,2}(58,:)'" : Constant  Value=[0.018719599069480126474207537512484122999012470245361328125;-0.031935339211156939243085872703886707313358783721923828125;0.0211159083844462309997869198241460253484547138214111328125;0.018524247199760847382155048990171053446829319000244140625;-0.021403635729746788018967862399222212843596935272216796875]
      mask Display: e = 0.06;c1 = [120 150 230]/255;c2 = ([120 150 230]+0)/383;c3 = ([120 150 230]+128)/383;patch([0 1 1 0],[0 0 1 1],c1);patch([0 1 1 1-e 1-e 0+e],[0 0 1 1-e 0+e 0+e],c2);patch([0 0 1 1-e 0+e 0+e],[0 1 1 1-e 1-e 0+e],c3);plot([0 1 1 0 0],[0 0 1 1 0]);disp('Weights');
  "IW{1,2}(59,:)'" : Constant  Value=[0.00726000427523675571916950133299906156025826930999755859375;-0.0084502660128260853600323798673343844711780548095703125;0.03336170261864608577173640924229403026401996612548828125;0.033602057132679434559019426842496613971889019012451171875;-0.031470766097081180612260453699491336010396480560302734375]
      mask Display: e = 0.06;c1 = [120 150 230]/255;c2 = ([120 150 230]+0)/383;c3 = ([120 150 230]+128)/383;patch([0 1 1 0],[0 0 1 1],c1);patch([0 1 1 1-e 1-e 0+e],[0 0 1 1-e 0+e 0+e],c2);patch([0 0 1 1-e 0+e 0+e],[0 1 1 1-e 1-e 0+e],c3);plot([0 1 1 0 0],[0 0 1 1 0]);disp('Weights');
  "IW{1,2}(6,:)'" : Constant  Value=[0.009305839580145282285972285762909450568258762359619140625;-0.008912780064853353945153457971173338592052459716796875;0.032073460666443946720516322557159583084285259246826171875;0.032121914880843739636961942096604616381227970123291015625;-0.0303758994485665741180913101970872958190739154815673828125]
      mask Display: e = 0.06;c1 = [120 150 230]/255;c2 = ([120 150 230]+0)/383;c3 = ([120 150 230]+128)/383;patch([0 1 1 0],[0 0 1 1],c1);patch([0 1 1 1-e 1-e 0+e],[0 0 1 1-e 0+e 0+e],c2);patch([0 0 1 1-e 0+e 0+e],[0 1 1 1-e 1-e 0+e],c3);plot([0 1 1 0 0],[0 0 1 1 0]);disp('Weights');
  "IW{1,2}(60,:)'" : Constant  Value=[-0.02182785855140501052318313668365590274333953857421875;0.01504526949072566843756959542588447220623493194580078125;-0.02370091772450612366274214082295657135546207427978515625;-0.0228758222728323475092526706475837272591888904571533203125;0.023484882859593568527056817174525349400937557220458984375]
      mask Display: e = 0.06;c1 = [120 150 230]/255;c2 = ([120 150 230]+0)/383;c3 = ([120 150 230]+128)/383;patch([0 1 1 0],[0 0 1 1],c1);patch([0 1 1 1-e 1-e 0+e],[0 0 1 1-e 0+e 0+e],c2);patch([0 0 1 1-e 0+e 0+e],[0 1 1 1-e 1-e 0+e],c3);plot([0 1 1 0 0],[0 0 1 1 0]);disp('Weights');
  "IW{1,2}(61,:)'" : Constant  Value=[-0.0257069752452846987667012257361420779488980770111083984375;0.033586657868722259723259782049353816546499729156494140625;-0.010764045820604174752421755556497373618185520172119140625;-0.007087499529581720199289396333597323973663151264190673828125;0.01164566976575382058201046930889788200147449970245361328125]
      mask Display: e = 0.06;c1 = [120 150 230]/255;c2 = ([120 150 230]+0)/383;c3 = ([120 150 230]+128)/383;patch([0 1 1 0],[0 0 1 1],c1);patch([0 1 1 1-e 1-e 0+e],[0 0 1 1-e 0+e 0+e],c2);patch([0 0 1 1-e 0+e 0+e],[0 1 1 1-e 1-e 0+e],c3);plot([0 1 1 0 0],[0 0 1 1 0]);disp('Weights');
  "IW{1,2}(62,:)'" : Constant  Value=[0.0078132320175603835188393730959433014504611492156982421875;-0.006626735256240343964473371585199856781400740146636962890625;0.03320555337067949974727554263154161162674427032470703125;0.033430740459620668370011031811372959055006504058837890625;-0.031321425335931241118458956407266668975353240966796875]
      mask Display: e = 0.06;c1 = [120 150 230]/255;c2 = ([120 150 230]+0)/383;c3 = ([120 150 230]+128)/383;patch([0 1 1 0],[0 0 1 1],c1);patch([0 1 1 1-e 1-e 0+e],[0 0 1 1-e 0+e 0+e],c2);patch([0 0 1 1-e 0+e 0+e],[0 1 1 1-e 1-e 0+e],c3);plot([0 1 1 0 0],[0 0 1 1 0]);disp('Weights');
  "IW{1,2}(63,:)'" : Constant  Value=[0.0251662608689834123298911805477473535574972629547119140625;-0.0164956603543140178924630845358478836715221405029296875;0.0199660386734384631690630840239464305341243743896484375;0.0181357705903712161654706136459935805760324001312255859375;-0.0197714541732280334185301029492620727978646755218505859375]
      mask Display: e = 0.06;c1 = [120 150 230]/255;c2 = ([120 150 230]+0)/383;c3 = ([120 150 230]+128)/383;patch([0 1 1 0],[0 0 1 1],c1);patch([0 1 1 1-e 1-e 0+e],[0 0 1 1-e 0+e 0+e],c2);patch([0 0 1 1-e 0+e 0+e],[0 1 1 1-e 1-e 0+e],c3);plot([0 1 1 0 0],[0 0 1 1 0]);disp('Weights');
  "IW{1,2}(64,:)'" : Constant  Value=[-0.0007413954615404926180854960904298422974534332752227783203125;0.033547985522193297935888978145158034749329090118408203125;-0.029191087786367857226377253709870274178683757781982421875;-0.0279593859396144485407464941317812190391123294830322265625;0.02850911114838171334096017517367727123200893402099609375]
      mask Display: e = 0.06;c1 = [120 150 230]/255;c2 = ([120 150 230]+0)/383;c3 = ([120 150 230]+128)/383;patch([0 1 1 0],[0 0 1 1],c1);patch([0 1 1 1-e 1-e 0+e],[0 0 1 1-e 0+e 0+e],c2);patch([0 0 1 1-e 0+e 0+e],[0 1 1 1-e 1-e 0+e],c3);plot([0 1 1 0 0],[0 0 1 1 0]);disp('Weights');
  "IW{1,2}(65,:)'" : Constant  Value=[-0.00981447060803192043720866166722771595232188701629638671875;0.00668974215954390612204338850688145612366497516632080078125;-0.031999750418018814424048201772166066803038120269775390625;-0.0321463622666899595525791255568037740886211395263671875;0.0301910869775281025251256750152606400661170482635498046875]
      mask Display: e = 0.06;c1 = [120 150 230]/255;c2 = ([120 150 230]+0)/383;c3 = ([120 150 230]+128)/383;patch([0 1 1 0],[0 0 1 1],c1);patch([0 1 1 1-e 1-e 0+e],[0 0 1 1-e 0+e 0+e],c2);patch([0 0 1 1-e 0+e 0+e],[0 1 1 1-e 1-e 0+e],c3);plot([0 1 1 0 0],[0 0 1 1 0]);disp('Weights');
  "IW{1,2}(66,:)'" : Constant  Value=[-0.00406862504623432645611824653997246059589087963104248046875;-0.029609417110996079369744649056883645243942737579345703125;0.031382930147386155217414938078945851884782314300537109375;0.0308010954472842206353089267167888465337455272674560546875;-0.0302090203856960858030955563435782096348702907562255859375]
      mask Display: e = 0.06;c1 = [120 150 230]/255;c2 = ([120 150 230]+0)/383;c3 = ([120 150 230]+128)/383;patch([0 1 1 0],[0 0 1 1],c1);patch([0 1 1 1-e 1-e 0+e],[0 0 1 1-e 0+e 0+e],c2);patch([0 0 1 1-e 0+e 0+e],[0 1 1 1-e 1-e 0+e],c3);plot([0 1 1 0 0],[0 0 1 1 0]);disp('Weights');
  "IW{1,2}(67,:)'" : Constant  Value=[0.0092045268860243244224417225041179335676133632659912109375;-0.0048143589814119980285767042005318216979503631591796875;0.032561046765026697979994452225582790561020374298095703125;0.03298507341447838581149909487066906876862049102783203125;-0.0306386907111728910846348838958874694071710109710693359375]
      mask Display: e = 0.06;c1 = [120 150 230]/255;c2 = ([120 150 230]+0)/383;c3 = ([120 150 230]+128)/383;patch([0 1 1 0],[0 0 1 1],c1);patch([0 1 1 1-e 1-e 0+e],[0 0 1 1-e 0+e 0+e],c2);patch([0 0 1 1-e 0+e 0+e],[0 1 1 1-e 1-e 0+e],c3);plot([0 1 1 0 0],[0 0 1 1 0]);disp('Weights');
  "IW{1,2}(68,:)'" : Constant  Value=[0.0166554445244073111298543921066084294579923152923583984375;0.0190564026610611225720504080527462065219879150390625;0.032175970339489205762628643014977569691836833953857421875;0.033420436026705226117972102883868501521646976470947265625;-0.0291330162573117563973301713531327550299465656280517578125]
      mask Display: e = 0.06;c1 = [120 150 230]/255;c2 = ([120 150 230]+0)/383;c3 = ([120 150 230]+128)/383;patch([0 1 1 0],[0 0 1 1],c1);patch([0 1 1 1-e 1-e 0+e],[0 0 1 1-e 0+e 0+e],c2);patch([0 0 1 1-e 0+e 0+e],[0 1 1 1-e 1-e 0+e],c3);plot([0 1 1 0 0],[0 0 1 1 0]);disp('Weights');
  "IW{1,2}(69,:)'" : Constant  Value=[-0.07933696170604050135199969417953980155289173126220703125;-0.09734733451014300487091901459280052222311496734619140625;0.00110657058715724477930553160121007749694399535655975341796875;0.00168109290085688011136266784006920715910382568836212158203125;-0.006049635266181991634371062360742143937386572360992431640625]
      mask Display: e = 0.06;c1 = [120 150 230]/255;c2 = ([120 150 230]+0)/383;c3 = ([120 150 230]+128)/383;patch([0 1 1 0],[0 0 1 1],c1);patch([0 1 1 1-e 1-e 0+e],[0 0 1 1-e 0+e 0+e],c2);patch([0 0 1 1-e 0+e 0+e],[0 1 1 1-e 1-e 0+e],c3);plot([0 1 1 0 0],[0 0 1 1 0]);disp('Weights');
  "IW{1,2}(7,:)'" : Constant  Value=[-0.00614442711631977590835962388382540666498243808746337890625;0.028867367052528847271020140397013165056705474853515625;-0.0291300358192916643285119704387398087419569492340087890625;-0.02757285715053804653340563390884199179708957672119140625;0.0283766277594770487124886670926571241579949855804443359375]
      mask Display: e = 0.06;c1 = [120 150 230]/255;c2 = ([120 150 230]+0)/383;c3 = ([120 150 230]+128)/383;patch([0 1 1 0],[0 0 1 1],c1);patch([0 1 1 1-e 1-e 0+e],[0 0 1 1-e 0+e 0+e],c2);patch([0 0 1 1-e 0+e 0+e],[0 1 1 1-e 1-e 0+e],c3);plot([0 1 1 0 0],[0 0 1 1 0]);disp('Weights');
  "IW{1,2}(70,:)'" : Constant  Value=[0.0112616053115305904397391856264221132732927799224853515625;0.01397049219305875229768520995321523514576256275177001953125;0.034488498786352815572708863101070164702832698822021484375;0.036036229241424633240598041084012947976589202880859375;-0.031514852860138879708795656142683583311736583709716796875]
      mask Display: e = 0.06;c1 = [120 150 230]/255;c2 = ([120 150 230]+0)/383;c3 = ([120 150 230]+128)/383;patch([0 1 1 0],[0 0 1 1],c1);patch([0 1 1 1-e 1-e 0+e],[0 0 1 1-e 0+e 0+e],c2);patch([0 0 1 1-e 0+e 0+e],[0 1 1 1-e 1-e 0+e],c3);plot([0 1 1 0 0],[0 0 1 1 0]);disp('Weights');
  "IW{1,2}(71,:)'" : Constant  Value=[-0.0132623586754215851135629833379425690509378910064697265625;0.002868393705742011169645966361940736533142626285552978515625;-0.0307533129975969023173210104005192988552153110504150390625;-0.0310004917439408826662639029336787643842399120330810546875;0.029023726793554201208724663274551858194172382354736328125]
      mask Display: e = 0.06;c1 = [120 150 230]/255;c2 = ([120 150 230]+0)/383;c3 = ([120 150 230]+128)/383;patch([0 1 1 0],[0 0 1 1],c1);patch([0 1 1 1-e 1-e 0+e],[0 0 1 1-e 0+e 0+e],c2);patch([0 0 1 1-e 0+e 0+e],[0 1 1 1-e 1-e 0+e],c3);plot([0 1 1 0 0],[0 0 1 1 0]);disp('Weights');
  "IW{1,2}(72,:)'" : Constant  Value=[0.0190645868575712203185634763258349266834557056427001953125;0.0189212830636668154216106785270312684588134288787841796875;0.0304246827780396654483663354540112777613103389739990234375;0.03144916659661479985121701474781730212271213531494140625;-0.0275619699311687345322230413557917927391827106475830078125]
      mask Display: e = 0.06;c1 = [120 150 230]/255;c2 = ([120 150 230]+0)/383;c3 = ([120 150 230]+128)/383;patch([0 1 1 0],[0 0 1 1],c1);patch([0 1 1 1-e 1-e 0+e],[0 0 1 1-e 0+e 0+e],c2);patch([0 0 1 1-e 0+e 0+e],[0 1 1 1-e 1-e 0+e],c3);plot([0 1 1 0 0],[0 0 1 1 0]);disp('Weights');
  "IW{1,2}(73,:)'" : Constant  Value=[0.01125137561491694297710619565577871981076896190643310546875;-0.005614051288826975467938229513720216345973312854766845703125;0.0309645340332998231236416586398263461887836456298828125;0.031287722150638332119232387640295200981199741363525390625;-0.0292710317298223270110479887762267026118934154510498046875]
      mask Display: e = 0.06;c1 = [120 150 230]/255;c2 = ([120 150 230]+0)/383;c3 = ([120 150 230]+128)/383;patch([0 1 1 0],[0 0 1 1],c1);patch([0 1 1 1-e 1-e 0+e],[0 0 1 1-e 0+e 0+e],c2);patch([0 0 1 1-e 0+e 0+e],[0 1 1 1-e 1-e 0+e],c3);plot([0 1 1 0 0],[0 0 1 1 0]);disp('Weights');
  "IW{1,2}(74,:)'" : Constant  Value=[-0.0168099108508360552127758325013928697444498538970947265625;-0.01232699033415462532004003293195637525059282779693603515625;-0.0310132526309297197608660923151546739973127841949462890625;-0.031992394206269640644091367676082882098853588104248046875;0.028539544550572552850109531163980136625468730926513671875]
      mask Display: e = 0.06;c1 = [120 150 230]/255;c2 = ([120 150 230]+0)/383;c3 = ([120 150 230]+128)/383;patch([0 1 1 0],[0 0 1 1],c1);patch([0 1 1 1-e 1-e 0+e],[0 0 1 1-e 0+e 0+e],c2);patch([0 0 1 1-e 0+e 0+e],[0 1 1 1-e 1-e 0+e],c3);plot([0 1 1 0 0],[0 0 1 1 0]);disp('Weights');
  "IW{1,2}(75,:)'" : Constant  Value=[0.024165027345370133915469779140039463527500629425048828125;-0.0271324359386713696851156640832414268516004085540771484375;0.014945167736129562341407250869451672770082950592041015625;0.01178533368410722252661582132304829428903758525848388671875;-0.01523385379494591497506750243928763666190207004547119140625]
      mask Display: e = 0.06;c1 = [120 150 230]/255;c2 = ([120 150 230]+0)/383;c3 = ([120 150 230]+128)/383;patch([0 1 1 0],[0 0 1 1],c1);patch([0 1 1 1-e 1-e 0+e],[0 0 1 1-e 0+e 0+e],c2);patch([0 0 1 1-e 0+e 0+e],[0 1 1 1-e 1-e 0+e],c3);plot([0 1 1 0 0],[0 0 1 1 0]);disp('Weights');
  "IW{1,2}(76,:)'" : Constant  Value=[0.017949411064963553819051611526447231881320476531982421875;-0.004558349088491485574803352420758528751321136951446533203125;0.0264987538001678103738445457793204695917665958404541015625;0.025930471364903777409249840957272681407630443572998046875;-0.025038910858188247188227393280612886883318424224853515625]
      mask Display: e = 0.06;c1 = [120 150 230]/255;c2 = ([120 150 230]+0)/383;c3 = ([120 150 230]+128)/383;patch([0 1 1 0],[0 0 1 1],c1);patch([0 1 1 1-e 1-e 0+e],[0 0 1 1-e 0+e 0+e],c2);patch([0 0 1 1-e 0+e 0+e],[0 1 1 1-e 1-e 0+e],c3);plot([0 1 1 0 0],[0 0 1 1 0]);disp('Weights');
  "IW{1,2}(77,:)'" : Constant  Value=[-0.0152170598833727514775926437096131849102675914764404296875;0.00940505604452042398566646852486883290112018585205078125;-0.0273417538502255010046670946621816256083548069000244140625;-0.0265147126094672815066477511436460190452635288238525390625;0.025986139415845647959724118436497519724071025848388671875]
      mask Display: e = 0.06;c1 = [120 150 230]/255;c2 = ([120 150 230]+0)/383;c3 = ([120 150 230]+128)/383;patch([0 1 1 0],[0 0 1 1],c1);patch([0 1 1 1-e 1-e 0+e],[0 0 1 1-e 0+e 0+e],c2);patch([0 0 1 1-e 0+e 0+e],[0 1 1 1-e 1-e 0+e],c3);plot([0 1 1 0 0],[0 0 1 1 0]);disp('Weights');
  "IW{1,2}(78,:)'" : Constant  Value=[0.0270741865692830131762125489558457047678530216217041015625;0.039179015525287595733683332355212769471108913421630859375;0.0287599823174846357110023831182843423448503017425537109375;0.03109420233947877976188323145834146998822689056396484375;-0.0253105774236535678578530195181883755140006542205810546875]
      mask Display: e = 0.06;c1 = [120 150 230]/255;c2 = ([120 150 230]+0)/383;c3 = ([120 150 230]+128)/383;patch([0 1 1 0],[0 0 1 1],c1);patch([0 1 1 1-e 1-e 0+e],[0 0 1 1-e 0+e 0+e],c2);patch([0 0 1 1-e 0+e 0+e],[0 1 1 1-e 1-e 0+e],c3);plot([0 1 1 0 0],[0 0 1 1 0]);disp('Weights');
  "IW{1,2}(79,:)'" : Constant  Value=[0.002729806859497307079676087226971503696404397487640380859375;0.025116394193320894234755513707568752579391002655029296875;-0.035264503253576905128507945619276142679154872894287109375;-0.035085791559983668663758038519517867825925350189208984375;0.0338035663093358140773858622196712531149387359619140625]
      mask Display: e = 0.06;c1 = [120 150 230]/255;c2 = ([120 150 230]+0)/383;c3 = ([120 150 230]+128)/383;patch([0 1 1 0],[0 0 1 1],c1);patch([0 1 1 1-e 1-e 0+e],[0 0 1 1-e 0+e 0+e],c2);patch([0 0 1 1-e 0+e 0+e],[0 1 1 1-e 1-e 0+e],c3);plot([0 1 1 0 0],[0 0 1 1 0]);disp('Weights');
  "IW{1,2}(8,:)'" : Constant  Value=[0.025722856149393395763791403396680834703147411346435546875;-0.02591667472707392949615723409806378185749053955078125;0.0120899399346782142339318255608304752968251705169677734375;0.0089203415169359194514253630359235103242099285125732421875;-0.01248505157225232760354050043360985000617802143096923828125]
      mask Display: e = 0.06;c1 = [120 150 230]/255;c2 = ([120 150 230]+0)/383;c3 = ([120 150 230]+128)/383;patch([0 1 1 0],[0 0 1 1],c1);patch([0 1 1 1-e 1-e 0+e],[0 0 1 1-e 0+e 0+e],c2);patch([0 0 1 1-e 0+e 0+e],[0 1 1 1-e 1-e 0+e],c3);plot([0 1 1 0 0],[0 0 1 1 0]);disp('Weights');
  "IW{1,2}(80,:)'" : Constant  Value=[-0.008620266741087789785780159945716150104999542236328125;0.0234608524889528824441953247514902614057064056396484375;-0.0260720301598917798824306402138972771354019641876220703125;-0.024378262171659274837320907636240008287131786346435546875;0.025090235426154135212062357140894164331257343292236328125]
      mask Display: e = 0.06;c1 = [120 150 230]/255;c2 = ([120 150 230]+0)/383;c3 = ([120 150 230]+128)/383;patch([0 1 1 0],[0 0 1 1],c1);patch([0 1 1 1-e 1-e 0+e],[0 0 1 1-e 0+e 0+e],c2);patch([0 0 1 1-e 0+e 0+e],[0 1 1 1-e 1-e 0+e],c3);plot([0 1 1 0 0],[0 0 1 1 0]);disp('Weights');
  "IW{1,2}(81,:)'" : Constant  Value=[0.0037141812299080058205891230471706876414828002452850341796875;-0.0162328160683163739974599337756444583646953105926513671875;0.033364390383923726857151592639638693071901798248291015625;0.033574250253109082231528503825757070444524288177490234375;-0.031848538465452942702871297342426260001957416534423828125]
      mask Display: e = 0.06;c1 = [120 150 230]/255;c2 = ([120 150 230]+0)/383;c3 = ([120 150 230]+128)/383;patch([0 1 1 0],[0 0 1 1],c1);patch([0 1 1 1-e 1-e 0+e],[0 0 1 1-e 0+e 0+e],c2);patch([0 0 1 1-e 0+e 0+e],[0 1 1 1-e 1-e 0+e],c3);plot([0 1 1 0 0],[0 0 1 1 0]);disp('Weights');
  "IW{1,2}(82,:)'" : Constant  Value=[-0.00910111983397448622012948504789164871908724308013916015625;-0.0189676834767861894615048612422469886951148509979248046875;-0.0368113692645511692003168491282849572598934173583984375;-0.038692040142375420941345254277621279470622539520263671875;0.033358575159280375033166166076625813730061054229736328125]
      mask Display: e = 0.06;c1 = [120 150 230]/255;c2 = ([120 150 230]+0)/383;c3 = ([120 150 230]+128)/383;patch([0 1 1 0],[0 0 1 1],c1);patch([0 1 1 1-e 1-e 0+e],[0 0 1 1-e 0+e 0+e],c2);patch([0 0 1 1-e 0+e 0+e],[0 1 1 1-e 1-e 0+e],c3);plot([0 1 1 0 0],[0 0 1 1 0]);disp('Weights');
  "IW{1,2}(83,:)'" : Constant  Value=[0.0145438971332256632151835873401068965904414653778076171875;0.002181532695806505210700532160217335331253707408905029296875;0.03072612084781096986052517650023219175636768341064453125;0.0310822059253560711855612908038892783224582672119140625;-0.0286747676289558044160354910445676068775355815887451171875]
      mask Display: e = 0.06;c1 = [120 150 230]/255;c2 = ([120 150 230]+0)/383;c3 = ([120 150 230]+128)/383;patch([0 1 1 0],[0 0 1 1],c1);patch([0 1 1 1-e 1-e 0+e],[0 0 1 1-e 0+e 0+e],c2);patch([0 0 1 1-e 0+e 0+e],[0 1 1 1-e 1-e 0+e],c3);plot([0 1 1 0 0],[0 0 1 1 0]);disp('Weights');
  "IW{1,2}(84,:)'" : Constant  Value=[-0.04636377237843769538727656254195608198642730712890625;0.007002741945924837417558617147506083711050450801849365234375;-0.006222546362353966083180711876821078476496040821075439453125;-0.0023856176565719179605284949730048538185656070709228515625;0.00671855657519706932212510963609020109288394451141357421875]
      mask Display: e = 0.06;c1 = [120 150 230]/255;c2 = ([120 150 230]+0)/383;c3 = ([120 150 230]+128)/383;patch([0 1 1 0],[0 0 1 1],c1);patch([0 1 1 1-e 1-e 0+e],[0 0 1 1-e 0+e 0+e],c2);patch([0 0 1 1-e 0+e 0+e],[0 1 1 1-e 1-e 0+e],c3);plot([0 1 1 0 0],[0 0 1 1 0]);disp('Weights');
  "IW{1,2}(85,:)'" : Constant  Value=[-0.01031882625643309493723709380219588638283312320709228515625;0.000709940638678782111846421454259825623012147843837738037109375;-0.032066981052519781536513931996523751877248287200927734375;-0.032331589597883007847212155638771946541965007781982421875;0.0298777587171027113333021674179690307937562465667724609375]
      mask Display: e = 0.06;c1 = [120 150 230]/255;c2 = ([120 150 230]+0)/383;c3 = ([120 150 230]+128)/383;patch([0 1 1 0],[0 0 1 1],c1);patch([0 1 1 1-e 1-e 0+e],[0 0 1 1-e 0+e 0+e],c2);patch([0 0 1 1-e 0+e 0+e],[0 1 1 1-e 1-e 0+e],c3);plot([0 1 1 0 0],[0 0 1 1 0]);disp('Weights');
  "IW{1,2}(86,:)'" : Constant  Value=[-0.01448235637275246782962323521815051208250224590301513671875;-0.01441100787924669453243797789809832465834915637969970703125;-0.033134057356373501634916323155266582034528255462646484375;-0.03445565569493864999106591540112276561558246612548828125;0.0303402395147106852812957100695712142623960971832275390625]
      mask Display: e = 0.06;c1 = [120 150 230]/255;c2 = ([120 150 230]+0)/383;c3 = ([120 150 230]+128)/383;patch([0 1 1 0],[0 0 1 1],c1);patch([0 1 1 1-e 1-e 0+e],[0 0 1 1-e 0+e 0+e],c2);patch([0 0 1 1-e 0+e 0+e],[0 1 1 1-e 1-e 0+e],c3);plot([0 1 1 0 0],[0 0 1 1 0]);disp('Weights');
  "IW{1,2}(87,:)'" : Constant  Value=[0.01168086656675894861867615048822699463926255702972412109375;0.0131453662947654988102375028802271117456257343292236328125;0.034427661524294154993253158636434818617999553680419921875;0.03625692962095004856504232293445966206490993499755859375;-0.031627494922346184591521733864283305592834949493408203125]
      mask Display: e = 0.06;c1 = [120 150 230]/255;c2 = ([120 150 230]+0)/383;c3 = ([120 150 230]+128)/383;patch([0 1 1 0],[0 0 1 1],c1);patch([0 1 1 1-e 1-e 0+e],[0 0 1 1-e 0+e 0+e],c2);patch([0 0 1 1-e 0+e 0+e],[0 1 1 1-e 1-e 0+e],c3);plot([0 1 1 0 0],[0 0 1 1 0]);disp('Weights');
  "IW{1,2}(88,:)'" : Constant  Value=[0.006548166009642357454634264968262868933379650115966796875;-0.006591367000971200436343355733015414443798363208770751953125;0.03367060253180716167253905268808011896908283233642578125;0.0338791920156046033607566414502798579633235931396484375;-0.031591745022834273604050991934855119325220584869384765625]
      mask Display: e = 0.06;c1 = [120 150 230]/255;c2 = ([120 150 230]+0)/383;c3 = ([120 150 230]+128)/383;patch([0 1 1 0],[0 0 1 1],c1);patch([0 1 1 1-e 1-e 0+e],[0 0 1 1-e 0+e 0+e],c2);patch([0 0 1 1-e 0+e 0+e],[0 1 1 1-e 1-e 0+e],c3);plot([0 1 1 0 0],[0 0 1 1 0]);disp('Weights');
  "IW{1,2}(89,:)'" : Constant  Value=[0.07890194809814458920538271513578365556895732879638671875;-0.02262703447011756019424666419581626541912555694580078125;-0.016677437490154829735633512655113008804619312286376953125;-0.022241977255538884772345653573211166076362133026123046875;0.01230072990948762046148345916662947274744510650634765625]
      mask Display: e = 0.06;c1 = [120 150 230]/255;c2 = ([120 150 230]+0)/383;c3 = ([120 150 230]+128)/383;patch([0 1 1 0],[0 0 1 1],c1);patch([0 1 1 1-e 1-e 0+e],[0 0 1 1-e 0+e 0+e],c2);patch([0 0 1 1-e 0+e 0+e],[0 1 1 1-e 1-e 0+e],c3);plot([0 1 1 0 0],[0 0 1 1 0]);disp('Weights');
  "IW{1,2}(9,:)'" : Constant  Value=[-0.01761818331388231850809233947074972093105316162109375;-0.03260752859142838910866402102328720502555370330810546875;0.043082051466879427159550886017314041964709758758544921875;0.043472200428442443753684898410938330926001071929931640625;-0.041063345467771850128002597557497210800647735595703125]
      mask Display: e = 0.06;c1 = [120 150 230]/255;c2 = ([120 150 230]+0)/383;c3 = ([120 150 230]+128)/383;patch([0 1 1 0],[0 0 1 1],c1);patch([0 1 1 1-e 1-e 0+e],[0 0 1 1-e 0+e 0+e],c2);patch([0 0 1 1-e 0+e 0+e],[0 1 1 1-e 1-e 0+e],c3);plot([0 1 1 0 0],[0 0 1 1 0]);disp('Weights');
  "IW{1,2}(90,:)'" : Constant  Value=[0.0310982729396096189977694024264565086923539638519287109375;0.036495139569617550401314787222872837446630001068115234375;0.0269681954699837779509952184753274195827543735504150390625;0.029450569366134403404000607906709774397313594818115234375;-0.024037929411202731133645471572890528477728366851806640625]
      mask Display: e = 0.06;c1 = [120 150 230]/255;c2 = ([120 150 230]+0)/383;c3 = ([120 150 230]+128)/383;patch([0 1 1 0],[0 0 1 1],c1);patch([0 1 1 1-e 1-e 0+e],[0 0 1 1-e 0+e 0+e],c2);patch([0 0 1 1-e 0+e 0+e],[0 1 1 1-e 1-e 0+e],c3);plot([0 1 1 0 0],[0 0 1 1 0]);disp('Weights');
  "IW{1,2}(91,:)'" : Constant  Value=[0.0141780065814262924706046220535426982678472995758056640625;0.01253158517431471503933426703270015423186123371124267578125;0.032662000333837253041036063905266928486526012420654296875;0.033903385237565288046202027771869325079023838043212890625;-0.03003482092008689929851783517733565531671047210693359375]
      mask Display: e = 0.06;c1 = [120 150 230]/255;c2 = ([120 150 230]+0)/383;c3 = ([120 150 230]+128)/383;patch([0 1 1 0],[0 0 1 1],c1);patch([0 1 1 1-e 1-e 0+e],[0 0 1 1-e 0+e 0+e],c2);patch([0 0 1 1-e 0+e 0+e],[0 1 1 1-e 1-e 0+e],c3);plot([0 1 1 0 0],[0 0 1 1 0]);disp('Weights');
  "IW{1,2}(92,:)'" : Constant  Value=[0.00847690551796616113822135929467549431137740612030029296875;-0.01154205384069932789625756441864723456092178821563720703125;0.03128096648504120891320923192324698902666568756103515625;0.031044791370552791975878648145226179622113704681396484375;-0.029662199269654708488896943663348793052136898040771484375]
      mask Display: e = 0.06;c1 = [120 150 230]/255;c2 = ([120 150 230]+0)/383;c3 = ([120 150 230]+128)/383;patch([0 1 1 0],[0 0 1 1],c1);patch([0 1 1 1-e 1-e 0+e],[0 0 1 1-e 0+e 0+e],c2);patch([0 0 1 1-e 0+e 0+e],[0 1 1 1-e 1-e 0+e],c3);plot([0 1 1 0 0],[0 0 1 1 0]);disp('Weights');
  "IW{1,2}(93,:)'" : Constant  Value=[-0.049940147318103610130091141172670177184045314788818359375;0.05305172997949121616034773296632920391857624053955078125;0.0001660949753107591694324673969873629175708629190921783447265625;0.00638094388765643970307106513928374624811112880706787109375;0.0036653012689656411411676106837376210023649036884307861328125]
      mask Display: e = 0.06;c1 = [120 150 230]/255;c2 = ([120 150 230]+0)/383;c3 = ([120 150 230]+128)/383;patch([0 1 1 0],[0 0 1 1],c1);patch([0 1 1 1-e 1-e 0+e],[0 0 1 1-e 0+e 0+e],c2);patch([0 0 1 1-e 0+e 0+e],[0 1 1 1-e 1-e 0+e],c3);plot([0 1 1 0 0],[0 0 1 1 0]);disp('Weights');
  "IW{1,2}(94,:)'" : Constant  Value=[-0.01647508129978826618700082917712279595434665679931640625;-0.0027389999995854376335646662710132659412920475006103515625;-0.029602333816844565717030235418860684148967266082763671875;-0.029942111247156129316682182661679689772427082061767578125;0.0277127828408428832085430570941753103397786617279052734375]
      mask Display: e = 0.06;c1 = [120 150 230]/255;c2 = ([120 150 230]+0)/383;c3 = ([120 150 230]+128)/383;patch([0 1 1 0],[0 0 1 1],c1);patch([0 1 1 1-e 1-e 0+e],[0 0 1 1-e 0+e 0+e],c2);patch([0 0 1 1-e 0+e 0+e],[0 1 1 1-e 1-e 0+e],c3);plot([0 1 1 0 0],[0 0 1 1 0]);disp('Weights');
  "IW{1,2}(95,:)'" : Constant  Value=[0.000131418039578988315140006815084916524938307702541351318359375;0.01547350982699500533679159985922524356283247470855712890625;-0.036357486905588314030079999383815447799861431121826171875;-0.036788589587290095039850967850725282914936542510986328125;0.034484970827406653814950487912938115186989307403564453125]
      mask Display: e = 0.06;c1 = [120 150 230]/255;c2 = ([120 150 230]+0)/383;c3 = ([120 150 230]+128)/383;patch([0 1 1 0],[0 0 1 1],c1);patch([0 1 1 1-e 1-e 0+e],[0 0 1 1-e 0+e 0+e],c2);patch([0 0 1 1-e 0+e 0+e],[0 1 1 1-e 1-e 0+e],c3);plot([0 1 1 0 0],[0 0 1 1 0]);disp('Weights');
  "IW{1,2}(96,:)'" : Constant  Value=[0.017896482798618919274336036551176221109926700592041015625;-0.0158092517903417016655875926289809285663068294525146484375;0.0128970969082707644093321874834146001376211643218994140625;0.0115924371183182724209803637904769857414066791534423828125;-0.01268912918113405431663753830662244581617414951324462890625]
      mask Display: e = 0.06;c1 = [120 150 230]/255;c2 = ([120 150 230]+0)/383;c3 = ([120 150 230]+128)/383;patch([0 1 1 0],[0 0 1 1],c1);patch([0 1 1 1-e 1-e 0+e],[0 0 1 1-e 0+e 0+e],c2);patch([0 0 1 1-e 0+e 0+e],[0 1 1 1-e 1-e 0+e],c3);plot([0 1 1 0 0],[0 0 1 1 0]);disp('Weights');
  "IW{1,2}(97,:)'" : Constant  Value=[-0.01241844602550823233044763327370674232952296733856201171875;0.026425275360450785344657020914382883347570896148681640625;-0.0228448209997699387685532457226145197637379169464111328125;-0.020785725592011992934882158579057431779801845550537109375;0.02234840554038765303435098985573858954012393951416015625]
      mask Display: e = 0.06;c1 = [120 150 230]/255;c2 = ([120 150 230]+0)/383;c3 = ([120 150 230]+128)/383;patch([0 1 1 0],[0 0 1 1],c1);patch([0 1 1 1-e 1-e 0+e],[0 0 1 1-e 0+e 0+e],c2);patch([0 0 1 1-e 0+e 0+e],[0 1 1 1-e 1-e 0+e],c3);plot([0 1 1 0 0],[0 0 1 1 0]);disp('Weights');
  "IW{1,2}(98,:)'" : Constant  Value=[0.0192097857861119360178836501518162549473345279693603515625;-0.01633009859141539010796151387694408185780048370361328125;0.0197190875645573727992232448968934477306902408599853515625;0.0178841220483899783488812573750692536123096942901611328125;-0.0190853557648222697806783543228448252193629741668701171875]
      mask Display: e = 0.06;c1 = [120 150 230]/255;c2 = ([120 150 230]+0)/383;c3 = ([120 150 230]+128)/383;patch([0 1 1 0],[0 0 1 1],c1);patch([0 1 1 1-e 1-e 0+e],[0 0 1 1-e 0+e 0+e],c2);patch([0 0 1 1-e 0+e 0+e],[0 1 1 1-e 1-e 0+e],c3);plot([0 1 1 0 0],[0 0 1 1 0]);disp('Weights');
  "IW{1,2}(99,:)'" : Constant  Value=[0.004415673281200388662626199476335386862047016620635986328125;0.046233443099180933366643131421369616873562335968017578125;-0.0306319019084238808314779589636600576341152191162109375;-0.0289246746044863577151939892928567132912576198577880859375;0.0304016958115495110337445083814600366167724132537841796875]
      mask Display: e = 0.06;c1 = [120 150 230]/255;c2 = ([120 150 230]+0)/383;c3 = ([120 150 230]+128)/383;patch([0 1 1 0],[0 0 1 1],c1);patch([0 1 1 1-e 1-e 0+e],[0 0 1 1-e 0+e 0+e],c2);patch([0 0 1 1-e 0+e 0+e],[0 1 1 1-e 1-e 0+e],c3);plot([0 1 1 0 0],[0 0 1 1 0]);disp('Weights');
  Mux : Mux  Inputs=100
      mask Display: e = 0.06;c1 = [120 150 230]/255;c2 = ([120 150 230]+0)/383;c3 = ([120 150 230]+128)/383;patch([0 1 1 0],[0 0 1 1],c1);patch([0 1 1 1-e 1-e 0+e],[0 0 1 1-e 0+e 0+e],c2);patch([0 0 1 1-e 0+e 0+e],[0 1 1 1-e 1-e 0+e],c3);plot([0 1 1 0 0],[0 0 1 1 0]);disp('Mux');
  dotprod{1..100} (100 alike) : neural/Weight Functions/dotprod
  "iz{1,2}" : Outport
      mask Display: e = 0.06;c1 = [120 230 180]/255;c2 = ([120 230 180]+0)/(256+128);c3 = ([120 230 180]+128)/(256+128);patch([0 1 1 0],[0 0 1 1],c1);patch([0 1 1 1-e 1-e 0+e],[0 0 1 1-e 0+e 0+e],c2);patch([0 0 1 1-e 0+e 0+e],[0 1 1 1-e 1-e 0+e],c3);plot([0 1 1 0 0],[0 0 1 1 0]);
  wires:
  Mux/1 -> "iz{1,2}"/1
  dotprod100/1 -> Mux/100
  "IW{1,2}(100,:)'"/1 -> dotprod100/1
  dotprod99/1 -> Mux/99
  "IW{1,2}(99,:)'"/1 -> dotprod99/1
  dotprod98/1 -> Mux/98
  "IW{1,2}(98,:)'"/1 -> dotprod98/1
  dotprod97/1 -> Mux/97
  "IW{1,2}(97,:)'"/1 -> dotprod97/1
  dotprod96/1 -> Mux/96
  "IW{1,2}(96,:)'"/1 -> dotprod96/1
  dotprod95/1 -> Mux/95
  "IW{1,2}(95,:)'"/1 -> dotprod95/1
  dotprod94/1 -> Mux/94
  "IW{1,2}(94,:)'"/1 -> dotprod94/1
  dotprod93/1 -> Mux/93
  "IW{1,2}(93,:)'"/1 -> dotprod93/1
  dotprod92/1 -> Mux/92
  "IW{1,2}(92,:)'"/1 -> dotprod92/1
  dotprod91/1 -> Mux/91
  "IW{1,2}(91,:)'"/1 -> dotprod91/1
  dotprod90/1 -> Mux/90
  "IW{1,2}(90,:)'"/1 -> dotprod90/1
  dotprod89/1 -> Mux/89
  "IW{1,2}(89,:)'"/1 -> dotprod89/1
  dotprod88/1 -> Mux/88
  "IW{1,2}(88,:)'"/1 -> dotprod88/1
  dotprod87/1 -> Mux/87
  "IW{1,2}(87,:)'"/1 -> dotprod87/1
  dotprod86/1 -> Mux/86
  "IW{1,2}(86,:)'"/1 -> dotprod86/1
  dotprod85/1 -> Mux/85
  "IW{1,2}(85,:)'"/1 -> dotprod85/1
  dotprod84/1 -> Mux/84
  "IW{1,2}(84,:)'"/1 -> dotprod84/1
  dotprod83/1 -> Mux/83
  "IW{1,2}(83,:)'"/1 -> dotprod83/1
  dotprod82/1 -> Mux/82
  "IW{1,2}(82,:)'"/1 -> dotprod82/1
  dotprod81/1 -> Mux/81
  "IW{1,2}(81,:)'"/1 -> dotprod81/1
  dotprod80/1 -> Mux/80
  "IW{1,2}(80,:)'"/1 -> dotprod80/1
  dotprod79/1 -> Mux/79
  "IW{1,2}(79,:)'"/1 -> dotprod79/1
  dotprod78/1 -> Mux/78
  "IW{1,2}(78,:)'"/1 -> dotprod78/1
  dotprod77/1 -> Mux/77
  "IW{1,2}(77,:)'"/1 -> dotprod77/1
  dotprod76/1 -> Mux/76
  "IW{1,2}(76,:)'"/1 -> dotprod76/1
  dotprod75/1 -> Mux/75
  "IW{1,2}(75,:)'"/1 -> dotprod75/1
  dotprod74/1 -> Mux/74
  "IW{1,2}(74,:)'"/1 -> dotprod74/1
  dotprod73/1 -> Mux/73
  "IW{1,2}(73,:)'"/1 -> dotprod73/1
  dotprod72/1 -> Mux/72
  "IW{1,2}(72,:)'"/1 -> dotprod72/1
  dotprod71/1 -> Mux/71
  "IW{1,2}(71,:)'"/1 -> dotprod71/1
  dotprod70/1 -> Mux/70
  "IW{1,2}(70,:)'"/1 -> dotprod70/1
  dotprod69/1 -> Mux/69
  "IW{1,2}(69,:)'"/1 -> dotprod69/1
  dotprod68/1 -> Mux/68
  "IW{1,2}(68,:)'"/1 -> dotprod68/1
  dotprod67/1 -> Mux/67
  "IW{1,2}(67,:)'"/1 -> dotprod67/1
  dotprod66/1 -> Mux/66
  "IW{1,2}(66,:)'"/1 -> dotprod66/1
  dotprod65/1 -> Mux/65
  "IW{1,2}(65,:)'"/1 -> dotprod65/1
  dotprod64/1 -> Mux/64
  "IW{1,2}(64,:)'"/1 -> dotprod64/1
  dotprod63/1 -> Mux/63
  "IW{1,2}(63,:)'"/1 -> dotprod63/1
  dotprod62/1 -> Mux/62
  "IW{1,2}(62,:)'"/1 -> dotprod62/1
  dotprod61/1 -> Mux/61
  "IW{1,2}(61,:)'"/1 -> dotprod61/1
  dotprod60/1 -> Mux/60
  "IW{1,2}(60,:)'"/1 -> dotprod60/1
  dotprod59/1 -> Mux/59
  "IW{1,2}(59,:)'"/1 -> dotprod59/1
  dotprod58/1 -> Mux/58
  "IW{1,2}(58,:)'"/1 -> dotprod58/1
  dotprod57/1 -> Mux/57
  "IW{1,2}(57,:)'"/1 -> dotprod57/1
  dotprod56/1 -> Mux/56
  "IW{1,2}(56,:)'"/1 -> dotprod56/1
  dotprod55/1 -> Mux/55
  "IW{1,2}(55,:)'"/1 -> dotprod55/1
  dotprod54/1 -> Mux/54
  "IW{1,2}(54,:)'"/1 -> dotprod54/1
  dotprod53/1 -> Mux/53
  "IW{1,2}(53,:)'"/1 -> dotprod53/1
  dotprod52/1 -> Mux/52
  "IW{1,2}(52,:)'"/1 -> dotprod52/1
  dotprod51/1 -> Mux/51
  "IW{1,2}(51,:)'"/1 -> dotprod51/1
  dotprod50/1 -> Mux/50
  "IW{1,2}(50,:)'"/1 -> dotprod50/1
  dotprod49/1 -> Mux/49
  "IW{1,2}(49,:)'"/1 -> dotprod49/1
  dotprod48/1 -> Mux/48
  "IW{1,2}(48,:)'"/1 -> dotprod48/1
  dotprod47/1 -> Mux/47
  "IW{1,2}(47,:)'"/1 -> dotprod47/1
  dotprod46/1 -> Mux/46
  "IW{1,2}(46,:)'"/1 -> dotprod46/1
  dotprod45/1 -> Mux/45
  "IW{1,2}(45,:)'"/1 -> dotprod45/1
  dotprod44/1 -> Mux/44
  "IW{1,2}(44,:)'"/1 -> dotprod44/1
  dotprod43/1 -> Mux/43
  "IW{1,2}(43,:)'"/1 -> dotprod43/1
  dotprod42/1 -> Mux/42
  "IW{1,2}(42,:)'"/1 -> dotprod42/1
  dotprod41/1 -> Mux/41
  "IW{1,2}(41,:)'"/1 -> dotprod41/1
  dotprod40/1 -> Mux/40
  "IW{1,2}(40,:)'"/1 -> dotprod40/1
  dotprod39/1 -> Mux/39
  "IW{1,2}(39,:)'"/1 -> dotprod39/1
  dotprod38/1 -> Mux/38
  "IW{1,2}(38,:)'"/1 -> dotprod38/1
  dotprod37/1 -> Mux/37
  "IW{1,2}(37,:)'"/1 -> dotprod37/1
  dotprod36/1 -> Mux/36
  "IW{1,2}(36,:)'"/1 -> dotprod36/1
  dotprod35/1 -> Mux/35
  "IW{1,2}(35,:)'"/1 -> dotprod35/1
  dotprod34/1 -> Mux/34
  "IW{1,2}(34,:)'"/1 -> dotprod34/1
  dotprod33/1 -> Mux/33
  "IW{1,2}(33,:)'"/1 -> dotprod33/1
  dotprod32/1 -> Mux/32
  "IW{1,2}(32,:)'"/1 -> dotprod32/1
  dotprod31/1 -> Mux/31
  "IW{1,2}(31,:)'"/1 -> dotprod31/1
  dotprod30/1 -> Mux/30
  "IW{1,2}(30,:)'"/1 -> dotprod30/1
  dotprod29/1 -> Mux/29
  "IW{1,2}(29,:)'"/1 -> dotprod29/1
  dotprod28/1 -> Mux/28
  "IW{1,2}(28,:)'"/1 -> dotprod28/1
  dotprod27/1 -> Mux/27
  "IW{1,2}(27,:)'"/1 -> dotprod27/1
  dotprod26/1 -> Mux/26
  "IW{1,2}(26,:)'"/1 -> dotprod26/1
  dotprod25/1 -> Mux/25
  "IW{1,2}(25,:)'"/1 -> dotprod25/1
  dotprod24/1 -> Mux/24
  "IW{1,2}(24,:)'"/1 -> dotprod24/1
  dotprod23/1 -> Mux/23
  "IW{1,2}(23,:)'"/1 -> dotprod23/1
  dotprod22/1 -> Mux/22
  "IW{1,2}(22,:)'"/1 -> dotprod22/1
  dotprod21/1 -> Mux/21
  "IW{1,2}(21,:)'"/1 -> dotprod21/1
  dotprod20/1 -> Mux/20
  "IW{1,2}(20,:)'"/1 -> dotprod20/1
  dotprod19/1 -> Mux/19
  "IW{1,2}(19,:)'"/1 -> dotprod19/1
  dotprod18/1 -> Mux/18
  "IW{1,2}(18,:)'"/1 -> dotprod18/1
  dotprod17/1 -> Mux/17
  "IW{1,2}(17,:)'"/1 -> dotprod17/1
  dotprod16/1 -> Mux/16
  "IW{1,2}(16,:)'"/1 -> dotprod16/1
  dotprod15/1 -> Mux/15
  "IW{1,2}(15,:)'"/1 -> dotprod15/1
  dotprod14/1 -> Mux/14
  "IW{1,2}(14,:)'"/1 -> dotprod14/1
  dotprod13/1 -> Mux/13
  "IW{1,2}(13,:)'"/1 -> dotprod13/1
  dotprod12/1 -> Mux/12
  "IW{1,2}(12,:)'"/1 -> dotprod12/1
  dotprod11/1 -> Mux/11
  "IW{1,2}(11,:)'"/1 -> dotprod11/1
  dotprod10/1 -> Mux/10
  "IW{1,2}(10,:)'"/1 -> dotprod10/1
  dotprod9/1 -> Mux/9
  "IW{1,2}(9,:)'"/1 -> dotprod9/1
  dotprod8/1 -> Mux/8
  "IW{1,2}(8,:)'"/1 -> dotprod8/1
  dotprod7/1 -> Mux/7
  "IW{1,2}(7,:)'"/1 -> dotprod7/1
  dotprod6/1 -> Mux/6
  "IW{1,2}(6,:)'"/1 -> dotprod6/1
  dotprod5/1 -> Mux/5
  "IW{1,2}(5,:)'"/1 -> dotprod5/1
  dotprod4/1 -> Mux/4
  "IW{1,2}(4,:)'"/1 -> dotprod4/1
  dotprod3/1 -> Mux/3
  "IW{1,2}(3,:)'"/1 -> dotprod3/1
  dotprod2/1 -> Mux/2
  "IW{1,2}(2,:)'"/1 -> dotprod2/1
  dotprod1/1 -> Mux/1
  "pd{1,2}"/1 -> dotprod100/2, dotprod99/2, dotprod98/2, dotprod97/2, dotprod96/2, dotprod95/2, dotprod94/2, dotprod93/2, dotprod92/2, dotprod91/2, dotprod90/2, dotprod89/2, dotprod88/2, dotprod87/2, dotprod86/2, dotprod85/2, dotprod84/2, dotprod83/2, dotprod82/2, dotprod81/2, dotprod80/2, dotprod79/2, dotprod78/2, dotprod77/2, dotprod76/2, dotprod75/2, dotprod74/2, dotprod73/2, dotprod72/2, dotprod71/2, dotprod70/2, dotprod69/2, dotprod68/2, dotprod67/2, dotprod66/2, dotprod65/2, dotprod64/2, dotprod63/2, dotprod62/2, dotprod61/2, dotprod60/2, dotprod59/2, dotprod58/2, dotprod57/2, dotprod56/2, dotprod55/2, dotprod54/2, dotprod53/2, dotprod52/2, dotprod51/2, dotprod50/2, dotprod49/2, dotprod48/2, dotprod47/2, dotprod46/2, dotprod45/2, dotprod44/2, dotprod43/2, dotprod42/2, dotprod41/2, dotprod40/2, dotprod39/2, dotprod38/2, dotprod37/2, dotprod36/2, dotprod35/2, dotprod34/2, dotprod33/2, dotprod32/2, dotprod31/2, dotprod30/2, dotprod29/2, dotprod28/2, dotprod27/2, dotprod26/2, dotprod25/2, dotprod24/2, dotprod23/2, dotprod22/2, dotprod21/2, dotprod20/2, dotprod19/2, dotprod18/2, dotprod17/2, dotprod16/2, dotprod15/2, dotprod14/2, dotprod13/2, dotprod12/2, dotprod11/2, dotprod10/2, dotprod9/2, dotprod8/2, dotprod7/2, dotprod6/2, dotprod5/2, dotprod4/2, dotprod3/2, dotprod2/2, dotprod1/2
  "IW{1,2}(1,:)'"/1 -> dotprod1/1
